simulink model "PandOAlgorithm"  (R2022b)
settings: Solver=ode23t  StartTime=0.0  StopTime=1  FixedStep=Ts_Power  RelTol=1e-7
undefined symbols (not defined in the file or in its folder): Cin, Cout, L, RL, Ts
libraries: simulink x6, spsSeriesRLCBranchLib x5, spsDiodeLib x3, spsPVArrayLib x3, spsCurrentMeasurementLib x2, spsMosfetLib x2, spsVoltageMeasurementLib x2, spsPWMGeneratorDCDCLib x1, spspowerguiLib x1
settings Model: SimulationMode=accelerator  Creator=MathWorks  LastModifiedBy=jfgf1
settings SolverCC: MaxConsecutiveZCs=1000000  ZeroCrossControl=EnableAll  AlgebraicLoopSolver=LineSearch
settings DataIOCC: LimitDataPoints=on  SaveFormat=Array  SignalLoggingSaveFormat=ModelDataLogs  ReturnWorkspaceOutputs=off
settings OptimizationCC: ExpressionDepthLimit=2147483647  LifeSpan=inf
settings DebuggingCC: UnderspecifiedInitializationDetection=Classic  MergeDetectMultiDrivingBlocksExec=none  SolverPrmCheckMsg=warning  FcnCallInpInsideContextMsg=warning  UnconnectedInputMsg=warning  UnconnectedOutputMsg=warning  UnconnectedLineMsg=warning  AllowSymbolicDim=off  StateNameClashWarn=warning  SFUnexpectedBacktrackingDiag=warning  SFNoUnconditionalDefaultTransitionDiag=warning  SFExecutionAtInitializationDiag=none  SFMachineParentedDataDiag=warning  ArithmeticOperatorsInVariantConditions=warning
settings HardwareCC: ProdBitPerPointer=32  ProdBitPerSizeT=32  ProdBitPerPtrDiffT=32  ProdLargestAtomicFloat=None  ProdIntDivRoundTo=Undefined  ProdEndianess=Unspecified  ProdWordSize=32  ProdHWDeviceType=32-bit Generic
settings ModelReferenceCC: EnableRefExpFcnMdlSchedulingChecks=on  PropagateSignalLabelsOutOfModel=off
settings SFSimCC: SimUseLocalCustomCode=off  CustomCodeUndefinedFunction=UseInterfaceOnly
settings RTWCC: RTWUseLocalCustomCode=off  DLArmComputeVersion=19.05
settings CodeAppCC: StateflowObjectComments=on
settings GRTTargetCC: TargetLangStandard=C89/C90 (ANSI)  CombineOutputUpdateFcns=off  GRTInterface=on
settings ConfigComp: CovMetricSettings=dw  CovSaveCumulativeToWorkspaceVar=on  CovSaveSingleToWorkspaceVar=on  CovExternalEMLEnable=off  CovSFcnEnable=off
settings SimscapeCC: SimscapeNormalizeSystem=off

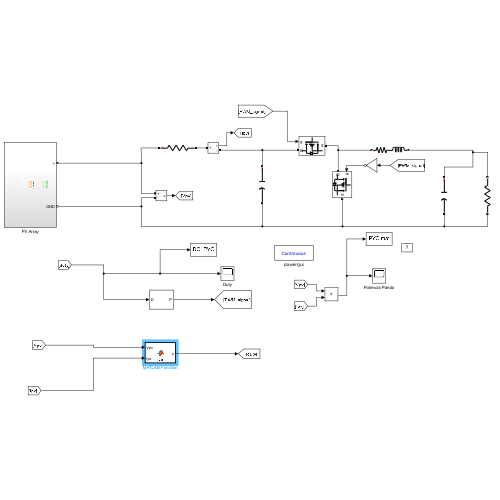
[thumbnail: Simulink's stored preview of the top-level diagram]
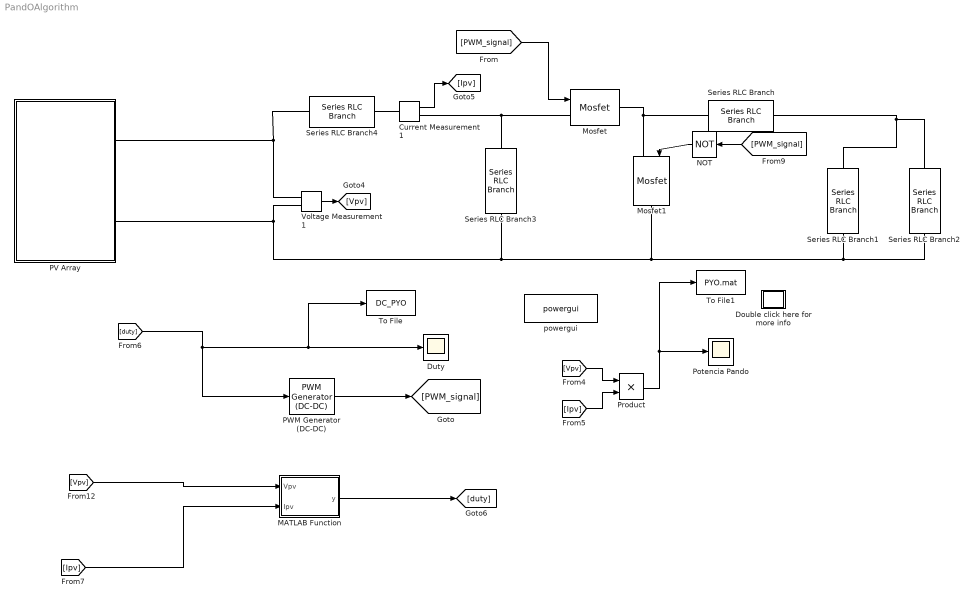
== system PandOAlgorithm ==
  Current Measurement1 : spsCurrentMeasurementLib/Current Measurement  PhasorSimulation=off  OutputType=Complex  PSBequivalent=0
  Double click here for more info : Subsystem
      settings: OpenFcn=showdemo(bdroot(gcb))
      mask Display: disp('?')
  Duty : Scope
  MATLAB Function : MATLAB Function  TreatAsAtomicUnit=on  SystemSampleTime=Ts
  Mosfet : spsMosfetLib/Mosfet  Ron=Ron  Lon=0  Rd=0.01  Vfd=0  IC=0  Rs=1e5  Cs=inf  Measurements=off
  Mosfet1 : spsMosfetLib/Mosfet  Ron=Ron  Lon=0  Rd=0.01  Vfd=0  IC=0  Rs=1e5  Cs=inf  Measurements=off
  NOT : Logic  Operator=NOT  IconShape=distinctive  AllPortsSameDT=off  OutDataTypeStr=boolean
  PV Array : Subsystem
  PWM Generator (DC-DC) : spsPWMGeneratorDCDCLib/PWM Generator (DC-DC)  Fsw=fs  Ts=0
  Potencia Pando : Scope
  Product : Product
  Series RLC Branch : spsSeriesRLCBranchLib/Series RLC Branch  LConnTagsString=__new0  RConnTagsString=__new0  BranchType=RL  Resistance=RL  Inductance=L  SetiL0=off  InitialCurrent=0  Capacitance=1e-6  Setx0=off  InitialVoltage=0  Measurements=None
  Series RLC Branch1 : spsSeriesRLCBranchLib/Series RLC Branch  LConnTagsString=__new0  RConnTagsString=__new0  BranchType=C  Resistance=0.005  Inductance=1e-3  SetiL0=off  InitialCurrent=0  Capacitance=Cout  Setx0=off  InitialVoltage=0  Measurements=None
  Series RLC Branch2 : spsSeriesRLCBranchLib/Series RLC Branch  LConnTagsString=__new0  RConnTagsString=__new0  BranchType=R  Resistance=1.1  Inductance=1e-3  SetiL0=off  InitialCurrent=0  Capacitance=1e-6  Setx0=off  InitialVoltage=0  Measurements=None
  Series RLC Branch3 : spsSeriesRLCBranchLib/Series RLC Branch  LConnTagsString=__new0  RConnTagsString=__new0  BranchType=C  Resistance=0.005  Inductance=1e-3  SetiL0=off  InitialCurrent=0  Capacitance=Cin  Setx0=off  InitialVoltage=0  Measurements=None
  Series RLC Branch4 : spsSeriesRLCBranchLib/Series RLC Branch  LConnTagsString=__new0  RConnTagsString=__new0  BranchType=R  Resistance=0.16  Inductance=1e-3  SetiL0=off  InitialCurrent=0  Capacitance=1e-6  Setx0=off  InitialVoltage=0  Measurements=None
  To File : ToFile  Filename=DC_PYO  SaveFormat=Timeseries  SampleTime=Ts
  To File1 : ToFile  Filename=PYO.mat  SaveFormat=Timeseries
  Voltage Measurement1 : spsVoltageMeasurementLib/Voltage Measurement  PhasorSimulation=off  OutputType=Complex  PSBequivalent=0
  powergui : spspowerguiLib/powergui  Priority=1  SimulationMode=Continuous  SampleTime=1e-06  frequency=60  Iterations=50  frequencyindice=0  Pbase=100e6  ErrMax=1e-4  UnitsV=kV  UnitsW=MW  buscounter=0  FunctionMessages=off  echomessages=off  EnableUseOfTLC=off  CurrentSourceSwitches=on  DisableSnubberDevices=on  DisableRonSwitches=off  DisableVfSwitches=off  DisplayEquations=off  AutomaticDiscreteSolvers=off  SolverType=Tustin/Backward Euler (TBE)  Interpol=off  ExternalGateDelay=off  methode=off  Ts=0  x0status=blocks  SPID=off  SwTol=0  HookPort=off  NonlinearTolerance=1e-4  nMaxIteration=100  ContinueOnMaxIteration=off  RestoreLinks=warning  ResistiveCurrentMeasurement=off  Frange=[0:2:500]  Ylog=off  Xlog=on  ShowGrid=off  save=off  variable=ZData  structure=0  ZoomFFT=on  StartTime=0.0  cycles=1  DisplayStyle=1  fundamental=60  FreqAxis=off  MaxFrequency=1000  frequencyindicesteady=1  RmsSteady=1  display=off
  wires:
  [PWM_signal] -> Mosfet/1
  Product/1 -> To File1/1, Potencia Pando/1
  [Ipv] -> Product/2
  [Vpv] -> Product/1
  Current Measurement1/1 -> [Ipv]
  MATLAB Function/1(y) -> [duty]
  NOT/1 -> Mosfet1/1
  [PWM_signal] -> NOT/1
  PWM Generator (DC-DC)/1 -> [PWM_signal]
  [duty] -> PWM Generator (DC-DC)/1, To File/1, Duty/1
  Voltage Measurement1/1 -> [Vpv]
  [Ipv] -> MATLAB Function/2(Ipv)
  [Vpv] -> MATLAB Function/1(Vpv)
  connections:
  Current Measurement1/RConn1 -- Series RLC Branch3/LConn1 -- Mosfet/LConn1
  Series RLC Branch2/RConn1 -- PV Array/RConn2 -- Voltage Measurement1/LConn2 -- Series RLC Branch3/RConn1 -- Mosfet1/RConn1 -- Series RLC Branch1/RConn1
  Series RLC Branch2/LConn1 -- Series RLC Branch/RConn1 -- Series RLC Branch1/LConn1
  PV Array/RConn1 -- Series RLC Branch4/LConn1 -- Voltage Measurement1/LConn1
  Series RLC Branch/LConn1 -- Mosfet1/LConn1 -- Mosfet/RConn1
  Current Measurement1/LConn1 -- Series RLC Branch4/RConn1

== system PandOAlgorithm/Double click here for more info ==

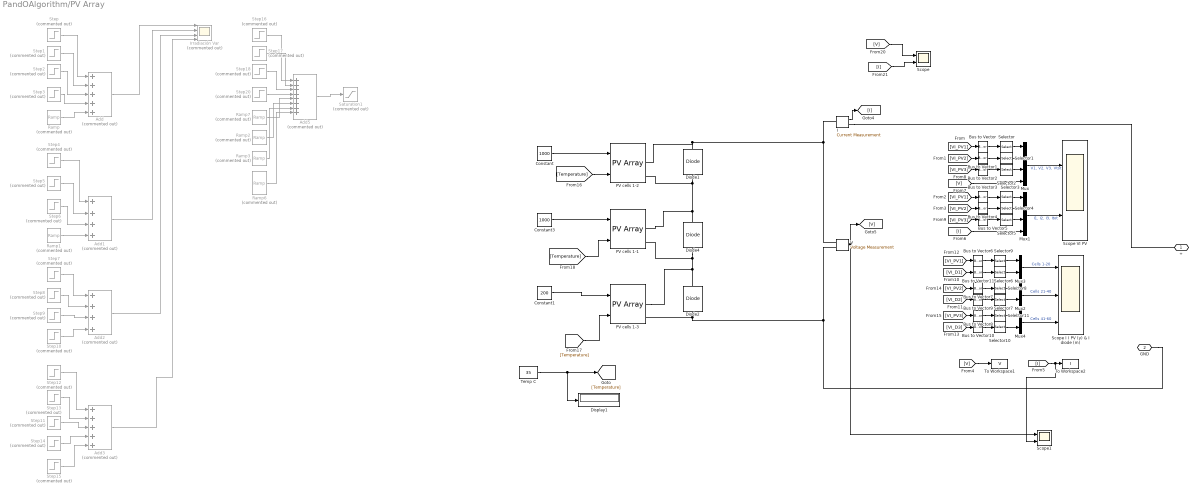
== system PandOAlgorithm/PV Array ==
  Add : Sum  Commented=on  Inputs=+++++
  Add1 : Sum  Commented=on  Inputs=++++
  Add2 : Sum  Commented=on  Inputs=++++
  Add3 : Sum  Commented=on  Inputs=+++++
  Add5 : Sum  Commented=on  Inputs=++++++++
  Bus to Vector{,1..11} (12 alike) : BusToVector
  Constant : Constant  Value=1000
  Constant1 : Constant  Value=200
  Constant3 : Constant  Value=1000
  Diode1 : spsDiodeLib/Diode  Ron=0.001  Lon=0  Vf=0.5  IC=0  UseSnubber=off  Rs=1e5*inf  Cs=inf  Measurements=off
  Diode2 : spsDiodeLib/Diode  Ron=0.001  Lon=0  Vf=0.5  IC=0  UseSnubber=off  Rs=1e5*inf  Cs=inf  Measurements=off
  Diode4 : spsDiodeLib/Diode  Ron=0.001  Lon=0  Vf=0.5  IC=0  UseSnubber=off  Rs=1e5*inf  Cs=inf  Measurements=off
  Display1 : Display
  I : spsCurrentMeasurementLib/Current Measurement  PhasorSimulation=off  OutputType=Complex  PSBequivalent=0
  Irradiación Var : Scope  Commented=on  NumInputPorts=4
  Mux : Mux
  Mux1 : Mux
  Mux2 : Mux  Inputs=2
  Mux3 : Mux  Inputs=2
  Mux4 : Mux  Inputs=2
  PV cells 1-1 : spsPVArrayLib/PV Array  Npar=1  Nser=1  PlotType=array @ 1000 W/m2 & specified temperatures  S_vec="[ 1000  500  100 ]"  Temp_C_vec=[ 20 ]  ModuleName=User-defined  PlotWhenSelected=off  Pm=83.83  Ncell=20  Voc=37.3/3  Isc=8.6  Vm=30.3/3  Im=8.3  beta_Voc_pc=-0.129  alpha_Isc_pc=0.044  beta_Voc=-0.016039  alpha_Isc=0.003784  IL=8.6716  I0=1.726e-15  nI=0.66942  Rsh=199.8499  Rs=0.14456  RobustModel=off  RobustCellTemperature=25  BAL=on  Tc=1e-5  Tfilter=5e-5
  PV cells 1-2 : spsPVArrayLib/PV Array  Npar=1  Nser=1  PlotType=array @ 1000 W/m2 & specified temperatures  S_vec="[ 1000  500  100 ]"  Temp_C_vec=[ 20 ]  ModuleName=User-defined  PlotWhenSelected=off  Pm=83.83  Ncell=20  Voc=37.3/3  Isc=8.6  Vm=30.3/3  Im=8.3  beta_Voc_pc=-0.129  alpha_Isc_pc=0.044  beta_Voc=-0.016039  alpha_Isc=0.003784  IL=8.6716  I0=1.726e-15  nI=0.66942  Rsh=199.8499  Rs=0.14456  RobustModel=off  RobustCellTemperature=25  BAL=on  Tc=1e-5  Tfilter=5e-5
  PV cells 1-3 : spsPVArrayLib/PV Array  Npar=1  Nser=1  PlotType=array @ 1000 W/m2 & specified temperatures  S_vec="[ 1000  500  100 ]"  Temp_C_vec=[ 20 ]  ModuleName=User-defined  PlotWhenSelected=off  Pm=83.83  Ncell=20  Voc=37.3/3  Isc=8.6  Vm=30.3/3  Im=8.3  beta_Voc_pc=-0.129  alpha_Isc_pc=0.044  beta_Voc=-0.016039  alpha_Isc=0.003784  IL=8.6716  I0=1.726e-15  nI=0.66942  Rsh=199.8499  Rs=0.14456  RobustModel=off  RobustCellTemperature=25  BAL=on  Tc=1e-5  Tfilter=5e-5
  Ramp : simulink/Sources/Ramp  Commented=on  slope=100  start=2.5  InitialOutput=0
  Ramp1 : simulink/Sources/Ramp  Commented=on  slope=100  start=2.5  InitialOutput=0
  Ramp2 : simulink/Sources/Ramp  Commented=on  slope=-100  start=5  InitialOutput=0
  Ramp3 : simulink/Sources/Ramp  Commented=on  slope=-100  start=6  InitialOutput=0
  Ramp6 : simulink/Sources/Ramp  Commented=on  slope=100  start=7  InitialOutput=0
  Ramp7 : simulink/Sources/Ramp  Commented=on  slope=100  start=2.5  InitialOutput=0
  Saturation1 : Saturate  Commented=on  UpperLimit=1000  LowerLimit=0
  Scope : Scope  NumInputPorts=2
  Scope I I PV (y) & I diode (m) : Scope  NumInputPorts=3
  Scope VI PV : Scope  NumInputPorts=2
  Scope1 : Scope  NumInputPorts=2
  Selector{,1..2,6..7,10} (6 alike) : Selector  InputPortWidth=2  IndexOptions=Index vector (dialog)  Indices=[1]  OutputSizes=1
  Selector{3..5,8..9,11} (6 alike) : Selector  InputPortWidth=2  IndexOptions=Index vector (dialog)  Indices=[2]  OutputSizes=1
  Step{,4,7,12,16} (5 alike) : Step  Commented=on  Time=0  After=1000  SampleTime=0
  Step1 : Step  Commented=on  After=-100  SampleTime=0
  Step10 : Step  Commented=on  Time=2  After=250  SampleTime=0
  Step11 : Step  Commented=on  After=100  SampleTime=0
  Step13 : Step  Commented=on  Time=0.5  After=-800  SampleTime=0
  Step14 : Step  Commented=on  Time=1.5  After=-200  SampleTime=0
  Step15 : Step  Commented=on  Time=2  After=200  SampleTime=0
  Step17 : Step  Commented=on  After=-100  SampleTime=0
  Step18 : Step  Commented=on  Time=1.5  After=-100  SampleTime=0
  Step2 : Step  Commented=on  Time=1.5  After=-100  SampleTime=0
  Step20 : Step  Commented=on  Time=2  After=-300  SampleTime=0
  Step3 : Step  Commented=on  Time=2  After=-300  SampleTime=0
  Step5 : Step  Commented=on  After=-100  SampleTime=0
  Step6 : Step  Commented=on  Time=1.5  After=-400  SampleTime=0
  Step8 : Step  Commented=on  After=-700  SampleTime=0
  Step9 : Step  Commented=on  Time=1.5  After=-150  SampleTime=0
  Temp C : Constant  Value=35
  To Workspace1 : ToWorkspace  VariableName=V  SampleTime=1e-3
  To Workspace2 : ToWorkspace  VariableName=I  SampleTime=1e-3
  V : spsVoltageMeasurementLib/Voltage Measurement  PhasorSimulation=off  OutputType=Complex  PSBequivalent=0
  + : PMIOPort  Side=Right
  GND : PMIOPort  Port=2  Side=Right
  wires:
  Mux/1 -> Scope VI PV/1  "V1, V2, V3, Vtot"
  [VI_PV3] -> Bus to Vector2/1
  Bus to Vector7/1 -> Selector8/1
  [VI_D1] -> Bus to Vector11/1
  Bus to Vector1/1 -> Selector1/1
  [VI_PV2] -> Bus to Vector4/1
  Selector4/1 -> Mux1/2
  Mux1/1 -> Scope VI PV/2  "I1, I2, I3, Itot"
  Mux4/1 -> Scope I I PV (y) & I diode (m)/3  "Cells 41-60"
  [VI_PV1] -> Bus to Vector6/1
  [VI_PV1] -> Bus to Vector3/1
  Selector3/1 -> Mux1/1
  Selector11/1 -> Mux4/1
  [V] -> Mux/4
  [V] -> To Workspace1/1
  Selector6/1 -> Mux3/2
  Selector/1 -> Mux/1
  Bus to Vector8/1 -> Selector11/1
  V/1 -> Scope1/1, [V]
  Mux2/1 -> Scope I I PV (y) & I diode (m)/2  "Cells 21-40"
  [I] -> Scope1/2, To Workspace2/1
  [VI_PV1] -> Bus to Vector/1
  Bus to Vector9/1 -> Selector7/1
  Selector5/1 -> Mux1/3
  [VI_PV2] -> Bus to Vector7/1
  [VI_PV3] -> Bus to Vector5/1
  I/1 -> [I]
  [VI_PV2] -> Bus to Vector1/1
  Selector8/1 -> Mux2/1
  [I] -> Mux1/4
  Bus to Vector4/1 -> Selector4/1
  Bus to Vector11/1 -> Selector6/1
  Selector2/1 -> Mux/3
  Bus to Vector10/1 -> Selector10/1
  Mux3/1 -> Scope I I PV (y) & I diode (m)/1  "Cells 1-20"
  Selector1/1 -> Mux/2
  Bus to Vector/1 -> Selector/1
  Bus to Vector6/1 -> Selector9/1
  Selector7/1 -> Mux2/2
  [VI_D2] -> Bus to Vector9/1
  [VI_PV3] -> Bus to Vector8/1
  Selector10/1 -> Mux4/2
  Bus to Vector2/1 -> Selector2/1
  Selector9/1 -> Mux3/1
  Bus to Vector3/1 -> Selector3/1
  Bus to Vector5/1 -> Selector5/1
  [VI_D3] -> Bus to Vector10/1
  Step1/1 -> Add/2
  Step/1 -> Add/1
  Ramp/1 -> Add/5
  Step3/1 -> Add/4
  Step2/1 -> Add/3
  Add3/1 -> Irradiación Var/4
  Add2/1 -> Irradiación Var/3
  Add1/1 -> Irradiación Var/2
  Add/1 -> Irradiación Var/1
  Temp C/1 -> [Temperature], Display1/1
  Step5/1 -> Add1/2
  Step4/1 -> Add1/1
  Ramp1/1 -> Add1/4
  Step6/1 -> Add1/3
  Step8/1 -> Add2/2
  Step9/1 -> Add2/3
  Step7/1 -> Add2/1
  Step10/1 -> Add2/4
  Step12/1 -> Add3/1
  Step13/1 -> Add3/2
  Step11/1 -> Add3/3
  Step14/1 -> Add3/4
  Step15/1 -> Add3/5
  [I] -> Scope/2
  [V] -> Scope/1
  [Temperature] -> PV cells 1-3/2
  [Temperature] -> PV cells 1-2/2
  [Temperature] -> PV cells 1-1/2
  Step17/1 -> Add5/2
  Ramp7/1 -> Add5/5
  Add5/1 -> Saturation1/1
  Ramp6/1 -> Add5/8
  Ramp2/1 -> Add5/6
  Step16/1 -> Add5/1
  Step18/1 -> Add5/3
  Step20/1 -> Add5/4
  Ramp3/1 -> Add5/7
  Constant/1 -> PV cells 1-2/1
  Constant3/1 -> PV cells 1-1/1
  Constant1/1 -> PV cells 1-3/1
  connections:
  Diode1/RConn1 -- PV cells 1-2/RConn1 -- I/LConn1 -- V/LConn1
  GND/RConn1 -- Diode2/LConn1 -- PV cells 1-3/RConn2 -- V/LConn2
  I/RConn1 -- +/RConn1
  Diode4/RConn1 -- PV cells 1-1/RConn1 -- PV cells 1-2/RConn2 -- Diode1/LConn1
  PV cells 1-1/RConn2 -- Diode4/LConn1 -- PV cells 1-3/RConn1 -- Diode2/RConn1

== matlab function PandOAlgorithm/MATLAB Function ==
  settings: updateMethod=DISCRETE
  data: Vpv input; y output; Ipv input
function y = fcn(Vpv, Ipv)

persistent Dprev Pprev Vprev

Ppv = Vpv*Ipv;

if isempty(Dprev)
    D = 0.2;
    Dprev = D;
    Vprev = Vpv;
    Pprev = Ppv;
    
else

deltaD = 0.03; %125e-6;

% Calculate measured array power
if (Ppv-Pprev)~= 0
    if (Ppv - Pprev) > 0
        if (Vpv - Vprev) > 0
            D = Dprev - deltaD;
        else
            D = Dprev + deltaD;
        end
    else
        if (Vpv-Vprev) > 0
            D = Dprev + deltaD;
        else
            D = Dprev - deltaD;
        end
    end
else
    D = Dprev;
end

if D < 0.15
    D = 0;
elseif D >0.9
    D = 1;
end
    
Dprev = D;
Vprev = Vpv;
Pprev = Ppv;
end

y = D;
